simulink model "test6"  (R2015a)
settings: Solver=ode45  StartTime=0.0  StopTime=480 * 640 + 100  RelTol=1e-3
InitFcn:
  | %% DSPBuilder Start
  | alt_dspbuilder_update_model(bdroot)
  | %% DSPBuilder End
libraries: allblocks_alteradspbuilder2 x37
settings Model: Creator=ASUS  LastModifiedBy=ASUS

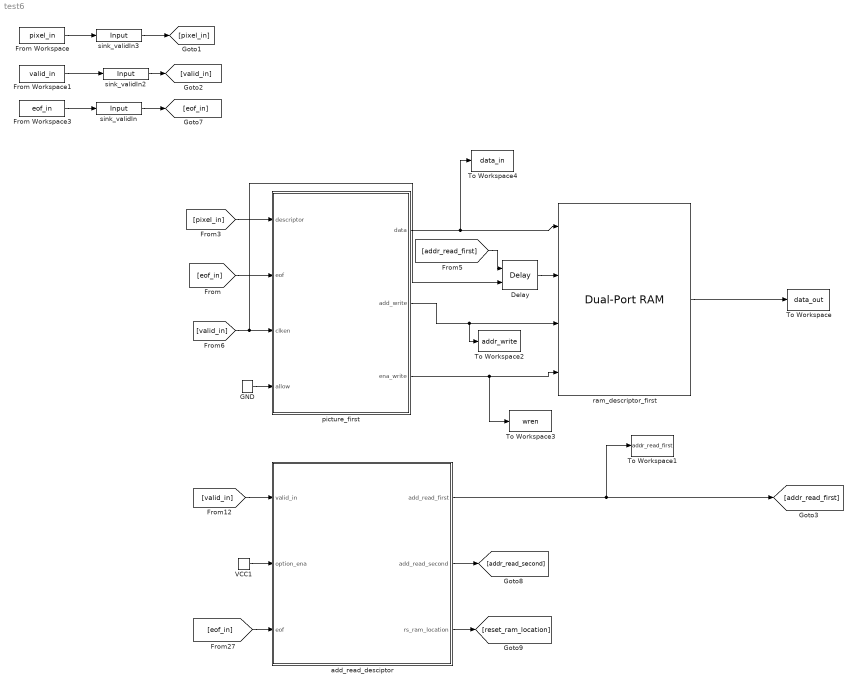
== system test6 ==
  Delay : allblocks_alteradspbuilder2/Delay  pipeline=2  pipeline_display=2  ClockPhase=1  use_ena=on  use_sclr=off  allowFloatingPointOverride=on  logOutputs=off  logFile=C:\Users\ASUS\Desktop\sift_fpga\Octave_2\tb_test6\test6_Delay.fixedpointlog  use_init=off  reset_value=1
  From Workspace : FromWorkspace  VariableName=pixel_in  SampleTime=0
  From Workspace1 : FromWorkspace  VariableName=valid_in  SampleTime=0
  From Workspace3 : FromWorkspace  VariableName=eof_in  SampleTime=0
  GND : allblocks_alteradspbuilder2/GND  SpecifyClock=off
  To Workspace : ToWorkspace  VariableName=data_out  SaveFormat=Timeseries  SampleTime=-1
  To Workspace1 : ToWorkspace  VariableName=addr_read_first  SaveFormat=Timeseries  SampleTime=-1
  To Workspace2 : ToWorkspace  VariableName=addr_write  SaveFormat=Timeseries  SampleTime=-1
  To Workspace3 : ToWorkspace  VariableName=wren  SaveFormat=Timeseries  SampleTime=-1
  To Workspace4 : ToWorkspace  VariableName=data_in  SaveFormat=Timeseries  SampleTime=-1
  VCC1 : allblocks_alteradspbuilder2/VCC  SpecifyClock=off
  add_read_desciptor : Subsystem
  picture_first : Subsystem
  ram_descriptor_first : allblocks_alteradspbuilder2/Dual-Port RAM  numwords=10000  BusType=Unsigned Integer  bwl=18  bwr=0  memory_type=AUTO  ram_type=DualRAM  dont_care=off  initialization=Blank  init_file=input.hex  init_array=[0:1:15]  register_outputs=on  use_ena=off  ClockPhase=1  allowFloatingPointOverride=on  logOutputs=off  logFile=C:\Users\ASUS\Desktop\sift_fpga\Octave_2\tb_test6\test6_ram%5Fdescriptor%5Ffirst.fixedpointlog  pipeline_display=2
  sink_validIn : allblocks_alteradspbuilder2/Input  iofile=C:\Users\ASUS\Desktop\sift_fpga\Octave_2\tb_test6\test6_sink%5FvalidIn.salt  BusType=Single Bit  bwl=8  bwr=0  SpecifyClock=off  PORTTYPE=Input  externalType=Inferred  allowFloatingPointOverride=on  logOutputs=off
  sink_validIn2 : allblocks_alteradspbuilder2/Input  iofile=C:\Users\ASUS\Desktop\sift_fpga\Octave_2\tb_test6\test6_sink%5FvalidIn2.salt  BusType=Single Bit  bwl=8  bwr=0  SpecifyClock=off  PORTTYPE=Input  externalType=Inferred  allowFloatingPointOverride=on  logOutputs=off
  sink_validIn3 : allblocks_alteradspbuilder2/Input  iofile=C:\Users\ASUS\Desktop\sift_fpga\Octave_2\tb_test6\test6_sink%5FvalidIn3.salt  BusType=Unsigned Integer  bwl=8  bwr=0  SpecifyClock=off  PORTTYPE=Input  externalType=Inferred  allowFloatingPointOverride=on  logOutputs=off
  wires:
  [pixel_in] -> picture_first/1(descriptor)
  picture_first/3(ena_write) -> To Workspace3/1, ram_descriptor_first/4
  [addr_read_first] -> Delay/1
  ram_descriptor_first/1 -> To Workspace/1
  [eof_in] -> picture_first/2(eof)
  [valid_in] -> Delay/2, picture_first/3(clken)
  From Workspace/1 -> sink_validIn3/1
  From Workspace3/1 -> sink_validIn/1
  From Workspace1/1 -> sink_validIn2/1
  sink_validIn/1 -> [eof_in]
  sink_validIn2/1 -> [valid_in]
  sink_validIn3/1 -> [pixel_in]
  [valid_in] -> add_read_desciptor/1(valid_in)
  VCC1/1 -> add_read_desciptor/2(option_ena)
  add_read_desciptor/1(add_read_first) -> To Workspace1/1, [addr_read_first]
  add_read_desciptor/2(add_read_second) -> [addr_read_second]
  add_read_desciptor/3(rs_ram_location) -> [reset_ram_location]
  [eof_in] -> add_read_desciptor/3(eof)
  GND/1 -> picture_first/4(allow)
  picture_first/2(add_write) -> To Workspace2/1, ram_descriptor_first/3
  picture_first/1(data) -> To Workspace4/1, ram_descriptor_first/1
  Delay/1 -> ram_descriptor_first/2

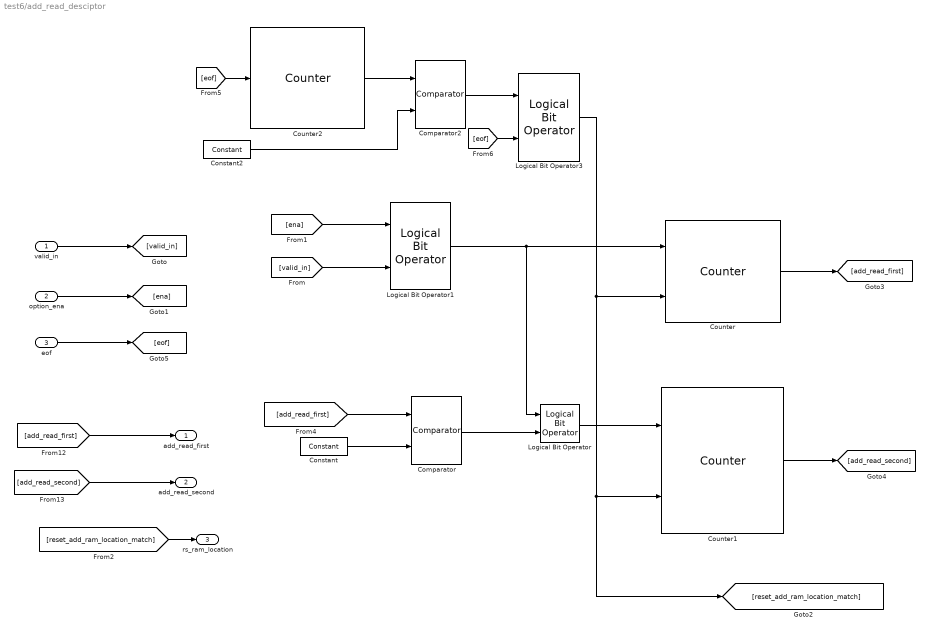
== system test6/add_read_desciptor ==
  valid_in : Inport
  option_ena : Inport  Port=2
  eof : Inport  Port=3
  Comparator : allblocks_alteradspbuilder2/Comparator  direction=a == b  pipeline_display=0  allowFloatingPointOverride=on  logOutputs=off  logFile=C:\Users\ASUS\Desktop\sift_fpga\Octave_2\tb_test6\test6_add%5Fread%5Fdesciptor_Comparator.fixedpointlog
  Comparator2 : allblocks_alteradspbuilder2/Comparator  direction=a == b  pipeline_display=0  allowFloatingPointOverride=on  logOutputs=off  logFile=C:\Users\ASUS\Desktop\sift_fpga\Octave_2\tb_test6\test6_add%5Fread%5Fdesciptor_Comparator2.fixedpointlog
  Constant : allblocks_alteradspbuilder2/Constant  mask_cst=999  BusType=Unsigned Integer  bwl=10  bwr=0  roundMode=Truncate  satMode=Wrap  SpecifyClock=off  allowFloatingPointOverride=on  logOutputs=off  logFile=C:\Users\ASUS\Desktop\sift_fpga\Octave_2\tb_test6\test6_add%5Fread%5Fdesciptor_Constant.fixedpointlog
  Constant2 : allblocks_alteradspbuilder2/Constant  mask_cst=2  BusType=Unsigned Integer  bwl=10  bwr=0  roundMode=Truncate  satMode=Wrap  SpecifyClock=off  allowFloatingPointOverride=on  logOutputs=off  logFile=C:\Users\ASUS\Desktop\sift_fpga\Octave_2\tb_test6\test6_add%5Fread%5Fdesciptor_Constant2.fixedpointlog
  Counter : allblocks_alteradspbuilder2/Counter  BusType=Unsigned Integer  bwl=10  bwr=0  use_modulo=on  modulo=1000  SpecifyClock=off  direction=Increment  use_sload=off  use_sset=off  svalue=1  use_clk_ena=off  use_ena=on  use_sclr=on  pipeline_display=1
  Counter1 : allblocks_alteradspbuilder2/Counter  BusType=Unsigned Integer  bwl=10  bwr=0  use_modulo=on  modulo=1000  SpecifyClock=off  direction=Increment  use_sload=off  use_sset=off  svalue=0  use_clk_ena=off  use_ena=on  use_sclr=on  pipeline_display=1
  Counter2 : allblocks_alteradspbuilder2/Counter  BusType=Unsigned Integer  bwl=2  bwr=0  use_modulo=on  modulo=3  SpecifyClock=off  direction=Increment  use_sload=off  use_sset=off  svalue=1  use_clk_ena=off  use_ena=on  use_sclr=off  pipeline_display=1
  Logical Bit Operator : allblocks_alteradspbuilder2/Logical Bit Operator  LogicalOperator=AND  user_inputs=2  pipeline_display=0
  Logical Bit Operator1 : allblocks_alteradspbuilder2/Logical Bit Operator  LogicalOperator=AND  user_inputs=2  pipeline_display=0
  Logical Bit Operator3 : allblocks_alteradspbuilder2/Logical Bit Operator  LogicalOperator=AND  user_inputs=2  pipeline_display=0
  add_read_first : Outport
  add_read_second : Outport  Port=2
  rs_ram_location : Outport  Port=3
  wires:
  Logical Bit Operator/1 -> Counter1/1
  [add_read_first] -> Comparator/1
  option_ena/1 -> [ena]
  Constant/1 -> Comparator/2
  Comparator/1 -> Logical Bit Operator/2
  valid_in/1 -> [valid_in]
  Counter1/1 -> [add_read_second]
  Counter/1 -> [add_read_first]
  Logical Bit Operator1/1 -> Logical Bit Operator/1, Counter/1
  [add_read_second] -> add_read_second/1
  [add_read_first] -> add_read_first/1
  [ena] -> Logical Bit Operator1/1
  [valid_in] -> Logical Bit Operator1/2
  [reset_add_ram_location_match] -> rs_ram_location/1
  [eof] -> Counter2/1
  Counter2/1 -> Comparator2/1
  Constant2/1 -> Comparator2/2
  eof/1 -> [eof]
  Logical Bit Operator3/1 -> [reset_add_ram_location_match], Counter1/2, Counter/2
  Comparator2/1 -> Logical Bit Operator3/1
  [eof] -> Logical Bit Operator3/2

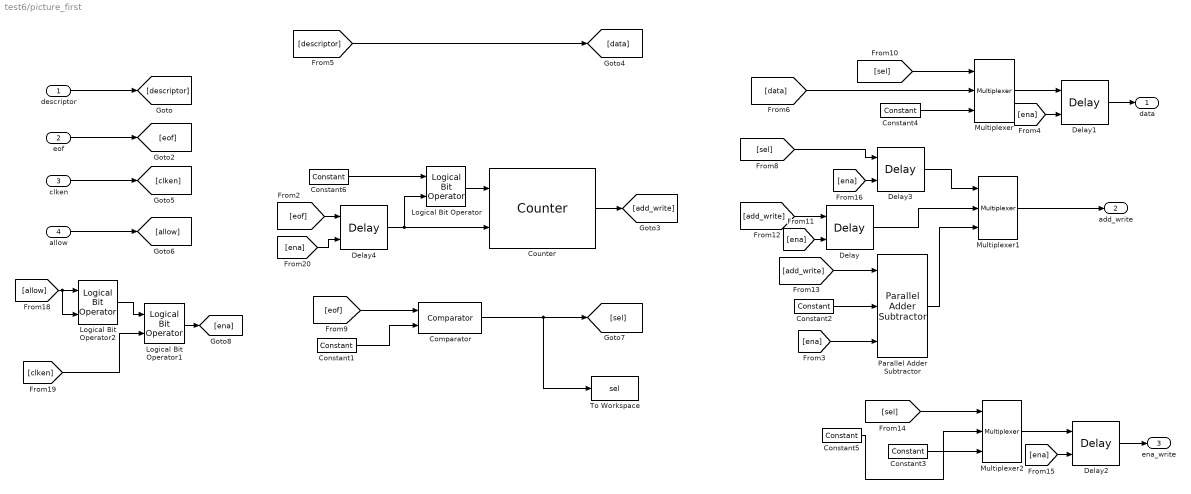
== system test6/picture_first ==
  descriptor : Inport
  eof : Inport  Port=2
  clken : Inport  Port=3
  allow : Inport  Port=4
  Comparator : allblocks_alteradspbuilder2/Comparator  direction=a == b  pipeline_display=0  allowFloatingPointOverride=on  logOutputs=off  logFile=C:\Users\ASUS\Desktop\sift_fpga\Octave_2\tb_test6\test6_picture%5Ffirst_Comparator.fixedpointlog
  Constant1 : allblocks_alteradspbuilder2/Constant  mask_cst=1  BusType=Single Bit  bwl=10  bwr=0  roundMode=Truncate  satMode=Wrap  SpecifyClock=off  allowFloatingPointOverride=on  logOutputs=off  logFile=C:\Users\ASUS\Desktop\sift_fpga\Octave_2\tb_test6\test6_picture%5Ffirst_Constant1.fixedpointlog
  Constant2 : allblocks_alteradspbuilder2/Constant  mask_cst=1  BusType=Unsigned Integer  bwl=10  bwr=0  roundMode=Truncate  satMode=Wrap  SpecifyClock=off  allowFloatingPointOverride=on  logOutputs=off  logFile=C:\Users\ASUS\Desktop\sift_fpga\Octave_2\tb_test6\test6_picture%5Ffirst_Constant2.fixedpointlog
  Constant3 : allblocks_alteradspbuilder2/Constant  mask_cst=1  BusType=Single Bit  bwl=1172  bwr=0  roundMode=Truncate  satMode=Wrap  SpecifyClock=off  allowFloatingPointOverride=on  logOutputs=off  logFile=C:\Users\ASUS\Desktop\sift_fpga\Octave_2\tb_test6\test6_picture%5Ffirst_Constant3.fixedpointlog
  Constant4 : allblocks_alteradspbuilder2/Constant  mask_cst=1098  BusType=Unsigned Integer  bwl=1172  bwr=0  roundMode=Truncate  satMode=Wrap  SpecifyClock=off  allowFloatingPointOverride=on  logOutputs=off  logFile=C:\Users\ASUS\Desktop\sift_fpga\Octave_2\tb_test6\test6_picture%5Ffirst_Constant4.fixedpointlog
  Constant5 : allblocks_alteradspbuilder2/Constant  mask_cst=1  BusType=Single Bit  bwl=1172  bwr=0  roundMode=Truncate  satMode=Wrap  SpecifyClock=off  allowFloatingPointOverride=on  logOutputs=off  logFile=C:\Users\ASUS\Desktop\sift_fpga\Octave_2\tb_test6\test6_picture%5Ffirst_Constant5.fixedpointlog
  Constant6 : allblocks_alteradspbuilder2/Constant  mask_cst=1  BusType=Single Bit  bwl=10  bwr=0  roundMode=Truncate  satMode=Wrap  SpecifyClock=off  allowFloatingPointOverride=on  logOutputs=off  logFile=C:\Users\ASUS\Desktop\sift_fpga\Octave_2\tb_test6\test6_picture%5Ffirst_Constant6.fixedpointlog
  Counter : allblocks_alteradspbuilder2/Counter  BusType=Unsigned Integer  bwl=10  bwr=0  use_modulo=on  modulo=1000  SpecifyClock=off  direction=Increment  use_sload=off  use_sset=off  svalue=1  use_clk_ena=off  use_ena=on  use_sclr=on  pipeline_display=1
  Delay : allblocks_alteradspbuilder2/Delay  pipeline=1  pipeline_display=1  ClockPhase=1  use_ena=on  use_sclr=off  allowFloatingPointOverride=on  logOutputs=off  logFile=C:\Users\ASUS\Desktop\sift_fpga\Octave_2\tb_test6\test6_picture%5Ffirst_Delay.fixedpointlog  use_init=off  reset_value=1
  Delay1 : allblocks_alteradspbuilder2/Delay  pipeline=1  pipeline_display=1  ClockPhase=1  use_ena=on  use_sclr=off  allowFloatingPointOverride=on  logOutputs=off  logFile=C:\Users\ASUS\Desktop\sift_fpga\Octave_2\tb_test6\test6_picture%5Ffirst_Delay1.fixedpointlog  use_init=off  reset_value=1
  Delay2 : allblocks_alteradspbuilder2/Delay  pipeline=1  pipeline_display=1  ClockPhase=1  use_ena=on  use_sclr=off  allowFloatingPointOverride=on  logOutputs=off  logFile=C:\Users\ASUS\Desktop\sift_fpga\Octave_2\tb_test6\test6_picture%5Ffirst_Delay2.fixedpointlog  use_init=off  reset_value=1
  Delay3 : allblocks_alteradspbuilder2/Delay  pipeline=1  pipeline_display=1  ClockPhase=1  use_ena=on  use_sclr=off  allowFloatingPointOverride=on  logOutputs=off  logFile=C:\Users\ASUS\Desktop\sift_fpga\Octave_2\tb_test6\test6_picture%5Ffirst_Delay3.fixedpointlog  use_init=off  reset_value=1
  Delay4 : allblocks_alteradspbuilder2/Delay  pipeline=1  pipeline_display=1  ClockPhase=1  use_ena=on  use_sclr=off  allowFloatingPointOverride=on  logOutputs=off  logFile=C:\Users\ASUS\Desktop\sift_fpga\Octave_2\tb_test6\test6_picture%5Ffirst_Delay4.fixedpointlog  use_init=off  reset_value=1
  Logical Bit Operator : allblocks_alteradspbuilder2/Logical Bit Operator  LogicalOperator=OR  user_inputs=2  pipeline_display=0
  Logical Bit Operator1 : allblocks_alteradspbuilder2/Logical Bit Operator  LogicalOperator=AND  user_inputs=2  pipeline_display=0
  Logical Bit Operator2 : allblocks_alteradspbuilder2/Logical Bit Operator  LogicalOperator=NAND  user_inputs=2  pipeline_display=0
  Multiplexer : allblocks_alteradspbuilder2/Multiplexer  numInputs=2  pipeline=0  oneHot=off  pipeline_display=0  use_ena=off  use_aclr=off  allowFloatingPointOverride=on  logOutputs=off  logFile=C:\Users\ASUS\Desktop\sift_fpga\Octave_2\tb_test6\test6_picture%5Ffirst_Multiplexer.fixedpointlog
  Multiplexer1 : allblocks_alteradspbuilder2/Multiplexer  numInputs=2  pipeline=0  oneHot=off  pipeline_display=0  use_ena=off  use_aclr=off  allowFloatingPointOverride=on  logOutputs=off  logFile=C:\Users\ASUS\Desktop\sift_fpga\Octave_2\tb_test6\test6_picture%5Ffirst_Multiplexer1.fixedpointlog
  Multiplexer2 : allblocks_alteradspbuilder2/Multiplexer  numInputs=2  pipeline=0  oneHot=off  pipeline_display=0  use_ena=off  use_aclr=off  allowFloatingPointOverride=on  logOutputs=off  logFile=C:\Users\ASUS\Desktop\sift_fpga\Octave_2\tb_test6\test6_picture%5Ffirst_Multiplexer2.fixedpointlog
  Parallel Adder Subtractor : allblocks_alteradspbuilder2/Parallel Adder Subtractor  number_of_inputs=2  direction=+  use_pipeline=on  pipeline_display=1  phase_selection=1  use_ena=on  use_aclr=off  allowFloatingPointOverride=on  logOutputs=off  logFile=C:\Users\ASUS\Desktop\sift_fpga\Octave_2\tb_test6\test6_picture%5Ffirst_Parallel+Adder+Subtractor.fixedpointlog
  To Workspace : ToWorkspace  VariableName=sel  SaveFormat=Timeseries  SampleTime=-1
  data : Outport
  add_write : Outport  Port=2
  ena_write : Outport  Port=3
  wires:
  descriptor/1 -> [descriptor]
  Constant6/1 -> Logical Bit Operator/1
  eof/1 -> [eof]
  [eof] -> Delay4/1
  Counter/1 -> [add_write]
  [descriptor] -> [data]
  [eof] -> Comparator/1
  Constant1/1 -> Comparator/2
  [sel] -> Multiplexer/1
  Multiplexer/1 -> Delay1/1
  Comparator/1 -> To Workspace/1, [sel]
  [data] -> Multiplexer/2
  Constant4/1 -> Multiplexer/3
  clken/1 -> [clken]
  Delay1/1 -> data/1
  [ena] -> Delay1/2
  [sel] -> Delay3/1
  [add_write] -> Delay/1
  Multiplexer1/1 -> add_write/1
  Delay/1 -> Multiplexer1/2
  [ena] -> Delay/2
  [add_write] -> Parallel Adder Subtractor/1
  Constant2/1 -> Parallel Adder Subtractor/2
  [ena] -> Parallel Adder Subtractor/3
  Parallel Adder Subtractor/1 -> Multiplexer1/3
  [sel] -> Multiplexer2/1
  Multiplexer2/1 -> Delay2/1
  Constant5/1 -> Multiplexer2/2
  Constant3/1 -> Multiplexer2/3
  Delay2/1 -> ena_write/1
  [ena] -> Delay2/2
  Delay3/1 -> Multiplexer1/1
  [ena] -> Delay3/2
  Logical Bit Operator/1 -> Counter/1
  Delay4/1 -> Counter/2, Logical Bit Operator/2
  [ena] -> Delay4/2
  allow/1 -> [allow]
  [allow] -> Logical Bit Operator2/2, Logical Bit Operator2/1
  [clken] -> Logical Bit Operator1/2
  Logical Bit Operator2/1 -> Logical Bit Operator1/1
  Logical Bit Operator1/1 -> [ena]
